simulink model "ROBOT2"  (R2016b)
settings: Solver=VariableStepDiscrete  StartTime=0.0  StopTime=inf  MaxStep=0.2  RelTol=1e-3
StartFcn:
  | 1
values from neighbouring files (symbols this model uses):
  s = dk(1:3,2)    [ik6dof.m]
undefined symbols (not defined in the file or in its folder): Assem1, link0, link1, link2_475, link3_475, link4_475, link5_475, link6_475, RootGround, RootPart
libraries: mblibv1 x24, simulink x6
settings Model: Creator=thanh  LastModifiedBy=thanh
settings OptimizationCC: BlockReduction=off
settings SimMechanicsCC: VisOnUpdateDiagram=on  VisDuringSimulation=on

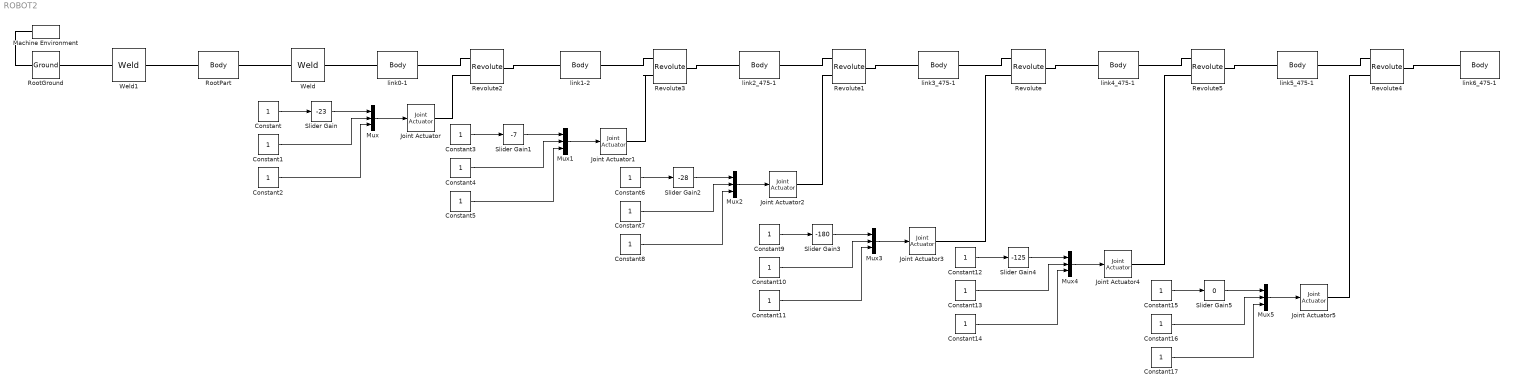
== system ROBOT2 ==
  Constant{,1..17} (18 alike) : Constant
  Joint Actuator{,1..5} (6 alike) : mblibv1/Sensors &  Actuators/Joint Actuator  UpdateFromCAD=off  PhysicalDomain=Mechanical  PortType=blob  ActuationStyle=Motion  AngleUnits=deg  ArcVelocityUnits=deg/s  ArcAccelerationUnits=deg/s^2  CoordPositionUnits=m  VelocityUnits=m/s  AccelerationUnits=m/s^2  ForceUnits=N  TorqueUnits=N*m  ActiveIO=on  Width=3  DialogClass=MechanicalActuatorBlock  Primitive=R1  ReferenceFrame=Absolute (World)
  Machine Environment : mblibv1/Bodies/Machine Environment  PortType=env  PhysicalDomain=Mechanical  DialogTemplateClass=MECH.MachineEnvironment  SyncWhenCopied=off  Gravity=[0 -9.81 0]  GravityUnits=m/s^2  GravityAsSignal=off  Dimensionality=Auto-detect  AnalysisType=Forward dynamics  LinearAssemblyTolerance=1e-3  LinearAssemblyToleranceUnits=m  AngularAssemblyTolerance=1e-3  AngularAssemblyToleranceUnits=rad  ConstraintSolverType=Stabilizing  ConstraintRelTolerance=1e-4  ConstraintAbsTolerance=1e-4  UseRobustSingularityHandling=off  RedundancyAnalysisToleranceType=Automatically select tolerance  RedundancyAnalysisTolerance=1e-14  StatePerturbationType=Fixed  PerturbationSize=1e-5  VisualizeMachine=on  BodyVisualizationType=Use model default body geometries  BodyColorSelMode=Use model default  DefaultBodyColor=[1 0 0]
  Mux{,1..5} (6 alike) : Mux  Inputs=3
  Revolute : mblibv1/Joints/Revolute  LConnTagsString=__newl0|SA1  RConnTagsString=__newr0  UpdateFromCAD=on  PMImportedID=link3_475-1:-:link4_475-1  NumSAPorts=1  CutJoint=off  MarkAsCut=off  Primitives=prismatic  PrimitiveProps=R1$World$[1,0,0]$revolute  DialogClass=JointBlock  R1Axis=[1,0,0]
  Revolute1 : mblibv1/Joints/Revolute  LConnTagsString=__newl0|SA1  RConnTagsString=__newr0  UpdateFromCAD=on  PMImportedID=link2_475-1:-:link3_475-1  NumSAPorts=1  CutJoint=off  MarkAsCut=off  Primitives=prismatic  PrimitiveProps=R1$World$[0,-1,0]$revolute  DialogClass=JointBlock  R1Axis=[0,-1,0]
  Revolute2 : mblibv1/Joints/Revolute  LConnTagsString=__newl0|SA1  RConnTagsString=__newr0  UpdateFromCAD=on  PMImportedID=link0-1:-:link1-2  NumSAPorts=1  CutJoint=off  MarkAsCut=off  Primitives=prismatic  PrimitiveProps=R1$World$[0,0,1]$revolute  DialogClass=JointBlock  R1Axis=[0,0,1]
  Revolute3 : mblibv1/Joints/Revolute  LConnTagsString=__newl0|SA1  RConnTagsString=__newr0  UpdateFromCAD=on  PMImportedID=link1-2:-:link2_475-1  NumSAPorts=1  CutJoint=off  MarkAsCut=off  Primitives=prismatic  PrimitiveProps=R1$World$[0,-1,0]$revolute  DialogClass=JointBlock  R1Axis=[0,-1,0]
  Revolute4 : mblibv1/Joints/Revolute  LConnTagsString=__newl0|SA1  RConnTagsString=__newr0  UpdateFromCAD=on  PMImportedID=link5_475-1:-:link6_475-1  NumSAPorts=1  CutJoint=off  MarkAsCut=off  Primitives=prismatic  PrimitiveProps=R1$World$[1,0,0]$revolute  DialogClass=JointBlock  R1Axis=[1,0,0]
  Revolute5 : mblibv1/Joints/Revolute  LConnTagsString=__newl0|SA1  RConnTagsString=__newr0  UpdateFromCAD=on  PMImportedID=link4_475-1:-:link5_475-1  NumSAPorts=1  CutJoint=off  MarkAsCut=off  Primitives=prismatic  PrimitiveProps=R1$World$[0,-1,0]$revolute  DialogClass=JointBlock  R1Axis=[0,-1,0]
  RootGround : mblibv1/Bodies/Ground  UpdateFromCAD=on  PMImportedID=RootGround  LeftPortType=env  RightPortType=workingframe  PhysicalDomain=Mechanical  DialogClass=GroundBlock  CoordPosition=[0.120011,-0.21352,0.614663]  CoordPositionUnits=m  StateVectorMgrId=1  MachineId=[2 0]  ShowEnvPort=on  ParameterChecksum=[683193410, 2989113359, 4181037304, 418117657]  TopologyChecksum=[1236414033, 3565595636, 815416478, 514460467]
  RootPart : mblibv1/Bodies/Body  LConnTagsString=CS3  RConnTagsString=CS2  UpdateFromCAD=on  PMImportedID=Assem1/RootPart  DialogClass=MechanicalBodyBlock  Mass=0  MassUnits=kg  InertiaUnits=kg*m^2  Inertia=[0,0,0;0,0,0;0,0,0]  Shape=Cylinder  ShapeDims=[1 1]  ShapeUnits=m  ShapeUse=false  Density=1  DensityUnits=kg/m^3  DensityUse=false  GraphicsMode=MACHINE_DEFAULT  BodyColorSelMode=MACHINE_DEFAULT  BodyColor=[1;0;0]  AttachedToCS=CS1  CG=Right$CG$[0.120011 -0.21352 0.614663]$WORLD$WORLD$m$[1 0 0;0 1 0;0 0 1]$3x3 Transform$rad$WORLD$false$Assem1/RootPart::CG(AUTOGEN)  WorkingFrames=Right$CS1$[0 0 0]$WORLD$WORLD$m$[1 0 0;0 1 0;0 0 1]$3x3 Transform$rad$WORLD$false$Assem1/RootPart::CS1(AUTOGEN)#Right$CS2$[0.0754243 -0.215 0.394926]$WORLD$WORLD$m$[1 0 0;0 1 0;0 0 1]$3x3 Transform$rad$WORLD$true$Assem1/RootPart:-:link0-1::Assem1/RootPart(AUTOGEN)#Left$CS3$[0.120011 -0.21352 0.614663]$WORLD$WORLD$m$[1 0 0;0 1 0;0 0 1]$3x3 Transform$rad$WORLD$true$Assem1/RootPart:-:RootGround::Assem1/RootPart(AUTOGEN)  CGPos=[0.120011 -0.21352 0.614663]  CGRot=[1 0 0;0 1 0;0 0 1]  CS0Pos=[]  CS0Rot=[]  CS1Pos=[0 0 0]  CS1Rot=[1 0 0;0 1 0;0 0 1]  CS2Pos=[0.0754243 -0.215 0.394926]  CS2Rot=[1 0 0;0 1 0;0 0 1]  CS3Pos=[0.120011 -0.21352 0.614663]  CS3Rot=[1 0 0;0 1 0;0 0 1]  CS4Pos=[]  CS4Rot=[]  CS5Pos=[]  CS5Rot=[]  CS6Pos=[]  CS6Rot=[]  CS7Pos=[]  CS7Rot=[]  CS8Pos=[]  CS8Rot=[]  CS9Pos=[]  CS9Rot=[]  CS10Pos=[]  CS10Rot=[]  CS11Pos=[]  CS11Rot=[]  CS12Pos=[]  CS12Rot=[]  CS13Pos=[]  CS13Rot=[]  CS14Pos=[]  CS14Rot=[]  CS15Pos=[]  CS15Rot=[]  CS16Pos=[]  CS16Rot=[]  CS17Pos=[]  CS17Rot=[]  CS18Pos=[]  CS18Rot=[]  CS19Pos=[]  CS19Rot=[]  CS20Pos=[]  CS20Rot=[]
  Slider Gain : simulink/Math Operations/Slider Gain  low=-230  gain=-23  high=230
  Slider Gain1 : simulink/Math Operations/Slider Gain  low=-115  gain=-7  high=113
  Slider Gain2 : simulink/Math Operations/Slider Gain  low=-205  gain=-28  high=55
  Slider Gain3 : simulink/Math Operations/Slider Gain  low=-230  gain=-180  high=230
  Slider Gain4 : simulink/Math Operations/Slider Gain  low=-125  gain=-125  high=120
  Slider Gain5 : simulink/Math Operations/Slider Gain  low=-400  gain=0  high=400
  Weld : mblibv1/Joints/Weld  LConnTagsString=__newl0  RConnTagsString=__newr0  UpdateFromCAD=on  PMImportedID=Assem1/RootPart:-:link0-1  NumSAPorts=0  CutJoint=off  MarkAsCut=off  Primitives=weld  PrimitiveProps=W$WORLD$[0.57735,0.57735,0.57735]$weld  DialogClass=JointBlock  WAxis=[0.57735,0.57735,0.57735]
  Weld1 : mblibv1/Joints/Weld  LConnTagsString=__newl0  RConnTagsString=__newr0  UpdateFromCAD=on  PMImportedID=Assem1/RootPart:-:RootGround  NumSAPorts=0  CutJoint=off  MarkAsCut=off  Primitives=weld  PrimitiveProps=W$WORLD$[0.57735,0.57735,0.57735]$weld  DialogClass=JointBlock  WAxis=[0.57735,0.57735,0.57735]
  link0-1 : mblibv1/Bodies/Body  LConnTagsString=CS2  RConnTagsString=CS3  UpdateFromCAD=on  PMImportedID=link0-1  DialogClass=MechanicalBodyBlock  Mass=3.54792  MassUnits=kg  InertiaUnits=kg*m^2  Inertia=[0.0112653,3.79287e-06,-7.63218e-05;3.79287e-06,0.0174774,3.68388e-08;-7.63218e-05,3.68388e-08,0.0149465]  Shape=Cylinder  ShapeDims=[1 1]  ShapeUnits=m  ShapeUse=false  Density=1  DensityUnits=kg/m^3  DensityUse=false  GraphicsMode=GFXFILE  GraphicsFileName=Assem1 - link0-1.STL  BodyColorSelMode=COLORPALETTE  BodyColor=[0.784314;0.8;0.788235]  AttachedToCS=CS1  CG=Right$CG$[0.0754243 -0.215 0.394926]$WORLD$WORLD$m$[1 0 0;0 1 0;0 0 1]$3x3 Transform$rad$WORLD$false$link0-1::CG(AUTOGEN)  WorkingFrames=Right$CS1$[0.103299 -0.215005 0.321045]$WORLD$WORLD$m$[1 0 0;0 1 0;0 0 1]$3x3 Transform$rad$WORLD$false$link0-1::CS1(AUTOGEN)#Left$CS2$[0.0754243 -0.215 0.394926]$WORLD$WORLD$m$[1 0 0;0 1 0;0 0 1]$3x3 Transform$rad$WORLD$true$Assem1/RootPart:-:link0-1::link0-1(AUTOGEN)#Right$CS3$[0.103299 -0.215005 0.494663]$WORLD$WORLD$m$[1 0 0;0 1 0;0 0 1]$3x3 Transform$rad$WORLD$true$link0-1:-:link1-2::link0-1(AUTOGEN)  CGPos=[0.0754243 -0.215 0.394926]  CGRot=[1 0 0;0 1 0;0 0 1]  CS0Pos=[]  CS0Rot=[]  CS1Pos=[0.103299 -0.215005 0.321045]  CS1Rot=[1 0 0;0 1 0;0 0 1]  CS2Pos=[0.0754243 -0.215 0.394926]  CS2Rot=[1 0 0;0 1 0;0 0 1]  CS3Pos=[0.103299 -0.215005 0.494663]  CS3Rot=[1 0 0;0 1 0;0 0 1]  CS4Pos=[]  CS4Rot=[]  CS5Pos=[]  CS5Rot=[]  CS6Pos=[]  CS6Rot=[]  CS7Pos=[]  CS7Rot=[]  CS8Pos=[]  CS8Rot=[]  CS9Pos=[]  CS9Rot=[]  CS10Pos=[]  CS10Rot=[]  CS11Pos=[]  CS11Rot=[]  CS12Pos=[]  CS12Rot=[]  CS13Pos=[]  CS13Rot=[]  CS14Pos=[]  CS14Rot=[]  CS15Pos=[]  CS15Rot=[]  CS16Pos=[]  CS16Rot=[]  CS17Pos=[]  CS17Rot=[]  CS18Pos=[]  CS18Rot=[]  CS19Pos=[]  CS19Rot=[]  CS20Pos=[]  CS20Rot=[]
  link1-2 : mblibv1/Bodies/Body  LConnTagsString=CS2  RConnTagsString=CS3  UpdateFromCAD=on  PMImportedID=link1-2  DialogClass=MechanicalBodyBlock  Mass=3.13079  MassUnits=kg  InertiaUnits=kg*m^2  Inertia=[0.0183498,1.20905e-05,0.000123573;1.20905e-05,0.0135287,-0.000121887;0.000123573,-0.000121887,0.0134462]  Shape=Cylinder  ShapeDims=[1 1]  ShapeUnits=m  ShapeUse=false  Density=1  DensityUnits=kg/m^3  DensityUse=false  GraphicsMode=GFXFILE  GraphicsFileName=Assem1 - link1-2.STL  BodyColorSelMode=COLORPALETTE  BodyColor=[0.784314;0.8;0.788235]  AttachedToCS=CS1  CG=Right$CG$[0.109586 -0.214529 0.556056]$WORLD$WORLD$m$[0.999391 -0.0348925 0;0.0348925 0.999391 0;0 0 1]$3x3 Transform$rad$WORLD$false$link1-2::CG(AUTOGEN)  WorkingFrames=Right$CS1$[0.103299 -0.215005 0.321545]$WORLD$WORLD$m$[0.999391 -0.0348925 0;0.0348925 0.999391 0;0 0 1]$3x3 Transform$rad$WORLD$false$link1-2::CS1(AUTOGEN)#Left$CS2$[0.103299 -0.215005 0.494663]$WORLD$WORLD$m$[1 0 0;0 1 0;0 0 1]$3x3 Transform$rad$WORLD$true$link0-1:-:link1-2::link1-2(AUTOGEN)#Right$CS3$[0.104904 -0.260977 0.648545]$WORLD$WORLD$m$[1 0 0;0 1 0;0 0 1]$3x3 Transform$rad$WORLD$true$link1-2:-:link2_475-1::link1-2(AUTOGEN)  CGPos=[0.109586 -0.214529 0.556056]  CGRot=[0.999391 -0.0348925 0;0.0348925 0.999391 0;0 0 1]  CS0Pos=[]  CS0Rot=[]  CS1Pos=[0.103299 -0.215005 0.321545]  CS1Rot=[0.999391 -0.0348925 0;0.0348925 0.999391 0;0 0 1]  CS2Pos=[0.103299 -0.215005 0.494663]  CS2Rot=[1 0 0;0 1 0;0 0 1]  CS3Pos=[0.104904 -0.260977 0.648545]  CS3Rot=[1 0 0;0 1 0;0 0 1]  CS4Pos=[]  CS4Rot=[]  CS5Pos=[]  CS5Rot=[]  CS6Pos=[]  CS6Rot=[]  CS7Pos=[]  CS7Rot=[]  CS8Pos=[]  CS8Rot=[]  CS9Pos=[]  CS9Rot=[]  CS10Pos=[]  CS10Rot=[]  CS11Pos=[]  CS11Rot=[]  CS12Pos=[]  CS12Rot=[]  CS13Pos=[]  CS13Rot=[]  CS14Pos=[]  CS14Rot=[]  CS15Pos=[]  CS15Rot=[]  CS16Pos=[]  CS16Rot=[]  CS17Pos=[]  CS17Rot=[]  CS18Pos=[]  CS18Rot=[]  CS19Pos=[]  CS19Rot=[]  CS20Pos=[]  CS20Rot=[]
  link2_475-1 : mblibv1/Bodies/Body  LConnTagsString=CS3  RConnTagsString=CS2  UpdateFromCAD=on  PMImportedID=link2_475-1  DialogClass=MechanicalBodyBlock  Mass=2.07438  MassUnits=kg  InertiaUnits=kg*m^2  Inertia=[0.0191337,-0.000102206,0.000122977;-0.000102206,0.0149555,6.46054e-05;0.000122977,6.46054e-05,0.00638626]  Shape=Cylinder  ShapeDims=[1 1]  ShapeUnits=m  ShapeUse=false  Density=1  DensityUnits=kg/m^3  DensityUse=false  GraphicsMode=GFXFILE  GraphicsFileName=Assem1 - link2_475-1.STL  BodyColorSelMode=COLORPALETTE  BodyColor=[0.792157;0.819608;0.933333]  AttachedToCS=CS1  CG=Right$CG$[0.0968485 -0.210905 0.747639]$WORLD$WORLD$m$[0.999136 -0.0348925 0.0225578;0.0348836 0.999391 0.000787578;-0.0225715 0 0.999745]$3x3 Transform$rad$WORLD$false$link2_475-1::CG(AUTOGEN)  WorkingFrames=Right$CS1$[0.0959579 -0.216262 0.321628]$WORLD$WORLD$m$[0.999136 -0.0348925 0.0225578;0.0348836 0.999391 0.000787578;-0.0225715 0 0.999745]$3x3 Transform$rad$WORLD$false$link2_475-1::CS1(AUTOGEN)#Right$CS2$[0.110102 -0.264298 0.873488]$WORLD$WORLD$m$[1 0 0;0 1 0;0 0 1]$3x3 Transform$rad$WORLD$true$link2_475-1:-:link3_475-1::link2_475-1(AUTOGEN)#Left$CS3$[0.104904 -0.260977 0.648545]$WORLD$WORLD$m$[1 0 0;0 1 0;0 0 1]$3x3 Transform$rad$WORLD$true$link1-2:-:link2_475-1::link2_475-1(AUTOGEN)  CGPos=[0.0968485 -0.210905 0.747639]  CGRot=[0.999136 -0.0348925 0.0225578;0.0348836 0.999391 0.000787578;-0.0225715 0 0.999745]  CS0Pos=[]  CS0Rot=[]  CS1Pos=[0.0959579 -0.216262 0.321628]  CS1Rot=[0.999136 -0.0348925 0.0225578;0.0348836 0.999391 0.000787578;-0.0225715 0 0.999745]  CS2Pos=[0.110102 -0.264298 0.873488]  CS2Rot=[1 0 0;0 1 0;0 0 1]  CS3Pos=[0.104904 -0.260977 0.648545]  CS3Rot=[1 0 0;0 1 0;0 0 1]  CS4Pos=[]  CS4Rot=[]  CS5Pos=[]  CS5Rot=[]  CS6Pos=[]  CS6Rot=[]  CS7Pos=[]  CS7Rot=[]  CS8Pos=[]  CS8Rot=[]  CS9Pos=[]  CS9Rot=[]  CS10Pos=[]  CS10Rot=[]  CS11Pos=[]  CS11Rot=[]  CS12Pos=[]  CS12Rot=[]  CS13Pos=[]  CS13Rot=[]  CS14Pos=[]  CS14Rot=[]  CS15Pos=[]  CS15Rot=[]  CS16Pos=[]  CS16Rot=[]  CS17Pos=[]  CS17Rot=[]  CS18Pos=[]  CS18Rot=[]  CS19Pos=[]  CS19Rot=[]  CS20Pos=[]  CS20Rot=[]
  link3_475-1 : mblibv1/Bodies/Body  LConnTagsString=CS3  RConnTagsString=CS2  UpdateFromCAD=on  PMImportedID=link3_475-1  DialogClass=MechanicalBodyBlock  Mass=1.0599  MassUnits=kg  InertiaUnits=kg*m^2  Inertia=[0.00156707,-9.96672e-06,-2.21656e-05;-9.96672e-06,0.00221805,-4.85618e-06;-2.21656e-05,-4.85618e-06,0.00187269]  Shape=Cylinder  ShapeDims=[1 1]  ShapeUnits=m  ShapeUse=false  Density=1  DensityUnits=kg/m^3  DensityUse=false  GraphicsMode=GFXFILE  GraphicsFileName=Assem1 - link3_475-1.STL  BodyColorSelMode=COLORPALETTE  BodyColor=[0.784314;0.8;0.788235]  AttachedToCS=CS1  CG=Right$CG$[0.099694 -0.215952 0.870391]$WORLD$WORLD$m$[0.999198 -0.0348925 0.0196587;0.0348858 0.999391 0.000686361;-0.0196707 0 0.999807]$3x3 Transform$rad$WORLD$false$link3_475-1::CG(AUTOGEN)  WorkingFrames=Right$CS1$[0.0975931 -0.217205 0.321594]$WORLD$WORLD$m$[0.999198 -0.0348925 0.0196587;0.0348858 0.999391 0.000686361;-0.0196707 0 0.999807]$3x3 Transform$rad$WORLD$false$link3_475-1::CS1(AUTOGEN)#Right$CS2$[0.181083 -0.21429 0.88206]$WORLD$WORLD$m$[1 0 0;0 1 0;0 0 1]$3x3 Transform$rad$WORLD$true$link3_475-1:-:link4_475-1::link3_475-1(AUTOGEN)#Left$CS3$[0.110102 -0.264298 0.873488]$WORLD$WORLD$m$[1 0 0;0 1 0;0 0 1]$3x3 Transform$rad$WORLD$true$link2_475-1:-:link3_475-1::link3_475-1(AUTOGEN)  CGPos=[0.099694 -0.215952 0.870391]  CGRot=[0.999198 -0.0348925 0.0196587;0.0348858 0.999391 0.000686361;-0.0196707 0 0.999807]  CS0Pos=[]  CS0Rot=[]  CS1Pos=[0.0975931 -0.217205 0.321594]  CS1Rot=[0.999198 -0.0348925 0.0196587;0.0348858 0.999391 0.000686361;-0.0196707 0 0.999807]  CS2Pos=[0.181083 -0.21429 0.88206]  CS2Rot=[1 0 0;0 1 0;0 0 1]  CS3Pos=[0.110102 -0.264298 0.873488]  CS3Rot=[1 0 0;0 1 0;0 0 1]  CS4Pos=[]  CS4Rot=[]  CS5Pos=[]  CS5Rot=[]  CS6Pos=[]  CS6Rot=[]  CS7Pos=[]  CS7Rot=[]  CS8Pos=[]  CS8Rot=[]  CS9Pos=[]  CS9Rot=[]  CS10Pos=[]  CS10Rot=[]  CS11Pos=[]  CS11Rot=[]  CS12Pos=[]  CS12Rot=[]  CS13Pos=[]  CS13Rot=[]  CS14Pos=[]  CS14Rot=[]  CS15Pos=[]  CS15Rot=[]  CS16Pos=[]  CS16Rot=[]  CS17Pos=[]  CS17Rot=[]  CS18Pos=[]  CS18Rot=[]  CS19Pos=[]  CS19Rot=[]  CS20Pos=[]  CS20Rot=[]
  link4_475-1 : mblibv1/Bodies/Body  LConnTagsString=CS2  RConnTagsString=CS3  UpdateFromCAD=on  PMImportedID=link4_475-1  DialogClass=MechanicalBodyBlock  Mass=1.2168  MassUnits=kg  InertiaUnits=kg*m^2  Inertia=[0.00178546,-5.47441e-05,0.000137546;-5.47441e-05,0.0040734,1.96232e-06;0.000137546,1.96232e-06,0.00446325]  Shape=Cylinder  ShapeDims=[1 1]  ShapeUnits=m  ShapeUse=false  Density=1  DensityUnits=kg/m^3  DensityUse=false  GraphicsMode=GFXFILE  GraphicsFileName=Assem1 - link4_475-1.STL  BodyColorSelMode=COLORPALETTE  BodyColor=[0.792157;0.819608;0.933333]  AttachedToCS=CS1  CG=Right$CG$[0.264604 -0.210791 0.883826]$WORLD$WORLD$m$[0.999198 -0.0354879 0.0185624;0.0348858 0.998885 0.0318126;-0.0196707 -0.0311395 0.999321]$3x3 Transform$rad$WORLD$false$link4_475-1::CG(AUTOGEN)  WorkingFrames=Right$CS1$[0.09721 -0.234733 0.321887]$WORLD$WORLD$m$[0.999198 -0.0354879 0.0185624;0.0348858 0.998885 0.0318126;-0.0196707 -0.0311395 0.999321]$3x3 Transform$rad$WORLD$false$link4_475-1::CS1(AUTOGEN)#Left$CS2$[0.181083 -0.21429 0.88206]$WORLD$WORLD$m$[1 0 0;0 1 0;0 0 1]$3x3 Transform$rad$WORLD$true$link3_475-1:-:link4_475-1::link4_475-1(AUTOGEN)#Right$CS3$[0.35863 -0.241596 0.879631]$WORLD$WORLD$m$[1 0 0;0 1 0;0 0 1]$3x3 Transform$rad$WORLD$true$link4_475-1:-:link5_475-1::link4_475-1(AUTOGEN)  CGPos=[0.264604 -0.210791 0.883826]  CGRot=[0.999198 -0.0354879 0.0185624;0.0348858 0.998885 0.0318126;-0.0196707 -0.0311395 0.999321]  CS0Pos=[]  CS0Rot=[]  CS1Pos=[0.09721 -0.234733 0.321887]  CS1Rot=[0.999198 -0.0354879 0.0185624;0.0348858 0.998885 0.0318126;-0.0196707 -0.0311395 0.999321]  CS2Pos=[0.181083 -0.21429 0.88206]  CS2Rot=[1 0 0;0 1 0;0 0 1]  CS3Pos=[0.35863 -0.241596 0.879631]  CS3Rot=[1 0 0;0 1 0;0 0 1]  CS4Pos=[]  CS4Rot=[]  CS5Pos=[]  CS5Rot=[]  CS6Pos=[]  CS6Rot=[]  CS7Pos=[]  CS7Rot=[]  CS8Pos=[]  CS8Rot=[]  CS9Pos=[]  CS9Rot=[]  CS10Pos=[]  CS10Rot=[]  CS11Pos=[]  CS11Rot=[]  CS12Pos=[]  CS12Rot=[]  CS13Pos=[]  CS13Rot=[]  CS14Pos=[]  CS14Rot=[]  CS15Pos=[]  CS15Rot=[]  CS16Pos=[]  CS16Rot=[]  CS17Pos=[]  CS17Rot=[]  CS18Pos=[]  CS18Rot=[]  CS19Pos=[]  CS19Rot=[]  CS20Pos=[]  CS20Rot=[]
  link5_475-1 : mblibv1/Bodies/Body  LConnTagsString=CS3  RConnTagsString=CS2  UpdateFromCAD=on  PMImportedID=link5_475-1  DialogClass=MechanicalBodyBlock  Mass=0.328496  MassUnits=kg  InertiaUnits=kg*m^2  Inertia=[0.000202405,7.47098e-06,4.00747e-09;7.47098e-06,0.000338242,-1.96019e-10;4.00747e-09,-1.96019e-10,0.000309042]  Shape=Cylinder  ShapeDims=[1 1]  ShapeUnits=m  ShapeUse=false  Density=1  DensityUnits=kg/m^3  DensityUse=false  GraphicsMode=GFXFILE  GraphicsFileName=Assem1 - link5_475-1.STL  BodyColorSelMode=COLORPALETTE  BodyColor=[0.792157;0.819608;0.933333]  AttachedToCS=CS1  CG=Right$CG$[0.370121 -0.206849 0.878398]$WORLD$WORLD$m$[0.999305 -0.0354879 0.0114008;0.0351129 0.998885 0.0315618;-0.0125082 -0.0311395 0.999437]$3x3 Transform$rad$WORLD$false$link5_475-1::CG(AUTOGEN)  WorkingFrames=Right$CS1$[0.101243 -0.235648 0.320062]$WORLD$WORLD$m$[0.999305 -0.0354879 0.0114008;0.0351129 0.998885 0.0315618;-0.0125082 -0.0311395 0.999437]$3x3 Transform$rad$WORLD$false$link5_475-1::CS1(AUTOGEN)#Right$CS2$[0.493029 -0.204369 0.876922]$WORLD$WORLD$m$[1 0 0;0 1 0;0 0 1]$3x3 Transform$rad$WORLD$true$link5_475-1:-:link6_475-1::link5_475-1(AUTOGEN)#Left$CS3$[0.35863 -0.241596 0.879631]$WORLD$WORLD$m$[1 0 0;0 1 0;0 0 1]$3x3 Transform$rad$WORLD$true$link4_475-1:-:link5_475-1::link5_475-1(AUTOGEN)  CGPos=[0.370121 -0.206849 0.878398]  CGRot=[0.999305 -0.0354879 0.0114008;0.0351129 0.998885 0.0315618;-0.0125082 -0.0311395 0.999437]  CS0Pos=[]  CS0Rot=[]  CS1Pos=[0.101243 -0.235648 0.320062]  CS1Rot=[0.999305 -0.0354879 0.0114008;0.0351129 0.998885 0.0315618;-0.0125082 -0.0311395 0.999437]  CS2Pos=[0.493029 -0.204369 0.876922]  CS2Rot=[1 0 0;0 1 0;0 0 1]  CS3Pos=[0.35863 -0.241596 0.879631]  CS3Rot=[1 0 0;0 1 0;0 0 1]  CS4Pos=[]  CS4Rot=[]  CS5Pos=[]  CS5Rot=[]  CS6Pos=[]  CS6Rot=[]  CS7Pos=[]  CS7Rot=[]  CS8Pos=[]  CS8Rot=[]  CS9Pos=[]  CS9Rot=[]  CS10Pos=[]  CS10Rot=[]  CS11Pos=[]  CS11Rot=[]  CS12Pos=[]  CS12Rot=[]  CS13Pos=[]  CS13Rot=[]  CS14Pos=[]  CS14Rot=[]  CS15Pos=[]  CS15Rot=[]  CS16Pos=[]  CS16Rot=[]  CS17Pos=[]  CS17Rot=[]  CS18Pos=[]  CS18Rot=[]  CS19Pos=[]  CS19Rot=[]  CS20Pos=[]  CS20Rot=[]
  link6_475-1 : mblibv1/Bodies/Body  LConnTagsString=CS2  UpdateFromCAD=on  PMImportedID=link6_475-1  DialogClass=MechanicalBodyBlock  Mass=0.00779756  MassUnits=kg  InertiaUnits=kg*m^2  Inertia=[1.7399e-06,6.09086e-10,3.60188e-11;6.09086e-10,8.9622e-07,-6.19783e-09;3.60188e-11,-6.19783e-09,9.32613e-07]  Shape=Cylinder  ShapeDims=[1 1]  ShapeUnits=m  ShapeUse=false  Density=1  DensityUnits=kg/m^3  DensityUse=false  GraphicsMode=GFXFILE  GraphicsFileName=Assem1 - link6_475-1.STL  BodyColorSelMode=COLORPALETTE  BodyColor=[0.792157;0.819608;0.933333]  AttachedToCS=CS1  CG=Right$CG$[0.417198 -0.20704 0.877807]$WORLD$WORLD$m$[0.999305 -0.0116149 0.0354184;0.0351129 0.612197 -0.789925;-0.0125082 0.79062 0.61218]$3x3 Transform$rad$WORLD$false$link6_475-1::CG(AUTOGEN)  WorkingFrames=Right$CS1$[0.0877456 0.226028 0.537701]$WORLD$WORLD$m$[0.999305 -0.0116149 0.0354184;0.0351129 0.612197 -0.789925;-0.0125082 0.79062 0.61218]$3x3 Transform$rad$WORLD$false$link6_475-1::CS1(AUTOGEN)#Left$CS2$[0.493029 -0.204369 0.876922]$WORLD$WORLD$m$[1 0 0;0 1 0;0 0 1]$3x3 Transform$rad$WORLD$true$link5_475-1:-:link6_475-1::link6_475-1(AUTOGEN)  CGPos=[0.417198 -0.20704 0.877807]  CGRot=[0.999305 -0.0116149 0.0354184;0.0351129 0.612197 -0.789925;-0.0125082 0.79062 0.61218]  CS0Pos=[]  CS0Rot=[]  CS1Pos=[0.0877456 0.226028 0.537701]  CS1Rot=[0.999305 -0.0116149 0.0354184;0.0351129 0.612197 -0.789925;-0.0125082 0.79062 0.61218]  CS2Pos=[0.493029 -0.204369 0.876922]  CS2Rot=[1 0 0;0 1 0;0 0 1]  CS3Pos=[]  CS3Rot=[]  CS4Pos=[]  CS4Rot=[]  CS5Pos=[]  CS5Rot=[]  CS6Pos=[]  CS6Rot=[]  CS7Pos=[]  CS7Rot=[]  CS8Pos=[]  CS8Rot=[]  CS9Pos=[]  CS9Rot=[]  CS10Pos=[]  CS10Rot=[]  CS11Pos=[]  CS11Rot=[]  CS12Pos=[]  CS12Rot=[]  CS13Pos=[]  CS13Rot=[]  CS14Pos=[]  CS14Rot=[]  CS15Pos=[]  CS15Rot=[]  CS16Pos=[]  CS16Rot=[]  CS17Pos=[]  CS17Rot=[]  CS18Pos=[]  CS18Rot=[]  CS19Pos=[]  CS19Rot=[]  CS20Pos=[]  CS20Rot=[]
  wires:
  Slider Gain/1 -> Mux/1
  Constant/1 -> Slider Gain/1
  Mux/1 -> Joint Actuator/1
  Constant1/1 -> Mux/2
  Constant2/1 -> Mux/3
  Slider Gain1/1 -> Mux1/1
  Constant3/1 -> Slider Gain1/1
  Mux1/1 -> Joint Actuator1/1
  Constant4/1 -> Mux1/2
  Constant5/1 -> Mux1/3
  Slider Gain2/1 -> Mux2/1
  Constant6/1 -> Slider Gain2/1
  Mux2/1 -> Joint Actuator2/1
  Constant7/1 -> Mux2/2
  Constant8/1 -> Mux2/3
  Slider Gain3/1 -> Mux3/1
  Constant9/1 -> Slider Gain3/1
  Mux3/1 -> Joint Actuator3/1
  Constant10/1 -> Mux3/2
  Constant11/1 -> Mux3/3
  Slider Gain4/1 -> Mux4/1
  Constant12/1 -> Slider Gain4/1
  Mux4/1 -> Joint Actuator4/1
  Constant13/1 -> Mux4/2
  Constant14/1 -> Mux4/3
  Slider Gain5/1 -> Mux5/1
  Constant15/1 -> Slider Gain5/1
  Mux5/1 -> Joint Actuator5/1
  Constant16/1 -> Mux5/2
  Constant17/1 -> Mux5/3
  connections:
  RootPart/RConn1 -- Weld/LConn1
  Weld/RConn1 -- link0-1/LConn1
  link3_475-1/RConn1 -- Revolute/LConn1
  Revolute/RConn1 -- link4_475-1/LConn1
  link2_475-1/RConn1 -- Revolute1/LConn1
  Revolute1/RConn1 -- link3_475-1/LConn1
  link0-1/RConn1 -- Revolute2/LConn1
  Revolute2/RConn1 -- link1-2/LConn1
  link1-2/RConn1 -- Revolute3/LConn1
  Revolute3/RConn1 -- link2_475-1/LConn1
  link5_475-1/RConn1 -- Revolute4/LConn1
  Revolute4/RConn1 -- link6_475-1/LConn1
  link4_475-1/RConn1 -- Revolute5/LConn1
  Revolute5/RConn1 -- link5_475-1/LConn1
  RootGround/RConn1 -- Weld1/LConn1
  Weld1/RConn1 -- RootPart/LConn1
  RootGround/LConn1 -- Machine Environment/RConn1
  Joint Actuator/RConn1 -- Revolute2/LConn2
  Revolute3/LConn2 -- Joint Actuator1/RConn1
  Joint Actuator2/RConn1 -- Revolute1/LConn2
  Joint Actuator3/RConn1 -- Revolute/LConn2
  Joint Actuator4/RConn1 -- Revolute5/LConn2
  Joint Actuator5/RConn1 -- Revolute4/LConn2
